simulink model "GNC2026W"  (R2024b)
settings: Solver=ode4  StartTime=0.0  StopTime=tsim  FixedStep=baseRate
values from neighbouring files (symbols this model uses):
  a = 1    [Run_Initializer.m]    (also in UKFoptimization.m)
  a1 = 0.236940    (= 0.23694)    [DrawARM.m]    (also in Run_Initializer.m = 2)
  a2 = 0.281536    [DrawARM.m]    (also in Run_Initializer.m = 2)
  a3 = 0.0621    [DrawARM.m]    (also in Run_Initializer.m = 2)
  A_c = eye(3)    [Run_Initializer.m]
  alpha = diag([a1; a2; a3])    [Run_Initializer.m]    (also in overlapping_trajectories.m = alpha_values1(ii); plotTrajectory.m = alpha_values(ii); plotfig.m = alpha_values(ii))
  b = 2    [Run_Initializer.m]    (also in UKFoptimization.m)
  b0 = 0.230400    (= 0.2304)    [DrawARM.m]
  b1 = 0.078980    (= 0.07898)    [DrawARM.m]
  b2 = 0.070384    [DrawARM.m]
  b3 = 0.070685    [DrawARM.m]
  CVrate = 1/5    (= 0.2)    [Run_Initializer.m]
  dt = baseRate    [Run_Initializer.m]    (also in UKFoptimization.m = 0.05; rms_plots.m = median(diff(tA)))
  F_u = zeros(3,1)    [Run_Initializer.m]
  fNum = 1    [Run_Initializer.m]
  gamma = r - (excess + shrink + bracketwidth)    (= 0.05023)    [DrawSpacecraft.m]    (also in Run_Initializer.m = diag([g1; g2; g3]))
  Gamma1_el = 0.12    [Run_Initializer.m]
  Gamma1_sh = 0.005    [Run_Initializer.m]
  Gamma1_wr = 0.025    [Run_Initializer.m]
  Gamma2_el = 5    [Run_Initializer.m]
  Gamma2_sh = 5    [Run_Initializer.m]
  Gamma2_wr = 5    [Run_Initializer.m]
  Gamma3_el = 10    [Run_Initializer.m]
  Gamma3_sh = 40    [Run_Initializer.m]
  Gamma3_wr = 40    [Run_Initializer.m]
  Gamma4_el = 0.039    [Run_Initializer.m]
  Gamma4_sh = 0.015    [Run_Initializer.m]
  Gamma4_wr = 0.029    [Run_Initializer.m]
  Gamma5_el = 800    [Run_Initializer.m]
  Gamma5_sh = 800    [Run_Initializer.m]
  Gamma5_wr = 800    [Run_Initializer.m]
  Gamma6_el = 0.000001    (= 1e-06)    [Run_Initializer.m]
  Gamma6_sh = 0.005    [Run_Initializer.m]
  Gamma6_wr = 0.02    [Run_Initializer.m]
  k = 5    [Run_Initializer.m]    (also in UKFoptimization.m)
  Kd_elarm = 0.8    [Run_Initializer.m]
  Kd_sharm = 1.0    (= 1)    [Run_Initializer.m]
  Kd_wrarm = 0.6    [Run_Initializer.m]
  Kp_elarm = 1.2    [Run_Initializer.m]
  Kp_sharm = 1.5    [Run_Initializer.m]
  Kp_wrarm = 1.0    (= 1)    [Run_Initializer.m]
  Mc_inv = inv(M_c)    [Run_Initializer.m]
  Phi = 73.2749*pi/180    (= 1.27888826407)    [DrawARM.m]
  PWMFreq = 5    [Run_Initializer.m]
  R = [cos(theta) -sin(theta) ... (first row only)    [Run_Initializer.m]    (also in UKFoptimization.m = diag([rx, rx, rt]))
  sep1 = 0.60    (= 0.6)    [Run_Initializer.m]
  sep2 = 0.30    (= 0.3)    [Run_Initializer.m]
  sep3 = 0.30    (= 0.3)    [Run_Initializer.m]
  Tz_lim_elarm = .1    (= 0.1)    [Run_Initializer.m]
  Tz_lim_sharm = .1    (= 0.1)    [Run_Initializer.m]
  Tz_lim_wrarm = .1    (= 0.1)    [Run_Initializer.m]
  VISinLoop = 1    [Run_Initializer.m]
  X1_blk = 0.4    [Run_Initializer.m]
  X2_blk = 0.4    [Run_Initializer.m]
  X3_blk = 0.4    [Run_Initializer.m]
  Y1_blk = 0.4    [Run_Initializer.m]
  Y2_blk = 0.4    [Run_Initializer.m]
  Y3_blk = 0.4    [Run_Initializer.m]
undefined symbols (not defined in the file or in its folder): baseRate, dataRate, DiscIntNeverNeededParam, drop_states_ARM, drop_states_BLACK, drop_states_BLUE, drop_states_RED, F_red_X_nominal, F_red_Y_nominal, F_thrusters_BLACK, F_thrusters_BLUE, F_thrusters_RED, home_states_BLACK, home_states_BLUE, home_states_RED, IBLACK, IBLUE, IDIST, IEE, init_states_BLACK, init_states_BLUE, init_states_RED, IPROX, IRED, K_BLACK, K_BLUE, K_RED, Kd_tb, Kd_tblue, Kd_tr, Kd_xb, Kd_xblue, Kd_xr, Kd_yb, Kd_yblue, Kd_yr, Kp_tb, Kp_tblue, Kp_tr, Kp_xb, Kp_xblue, Kp_xr, Kp_yb, Kp_yblue, Kp_yr, mBLACK, mBLUE, mDIST, mEE, mPROX, mRED, Phase0_End, Phase1_End, Phase2_End, Phase3_End, Phase3_SubPhase1_End, Phase3_SubPhase2_End, Phase3_SubPhase3_End, Phase3_SubPhase4_End, Phase4_End ... (+10)
libraries: simulink x30, nvidiaSharedBlocks x20, MainLibrary x5, dspinverses x3, commrandsrc3 x1, nvidiaIMUSensorslib x1
(part 8 of 9)

== matlab function GNC2026W/Simulate Plant Dynamics/RED and ARM Dynamics/RED + ARM/Coriolis Function1 ==
  data: a1 parameter; a2 parameter; a3 parameter; b0 parameter; b1 parameter; b2 parameter; mPROX parameter; mDIST parameter; mEE parameter; Phi parameter; CoriolisS output; x input
function CoriolisS = CoriolisFunc3LINK(a1,a2,a3,b0,b1,b2,mPROX,mDIST,mEE,Phi,x)
%CORIOLISFUNC3LINK
%    CORIOLISS = CORIOLISFUNC3LINK(A1,A2,A3,B0,B1,B2,mPROX,mDIST,mEE,PHI,Q0,Q1,Q2,Q3,Q0_DOT,Q1_DOT,Q2_DOT,Q3_DOT)

%    This function was generated by the Symbolic Math Toolbox version 8.0.
%    05-Nov-2017 11:48:44

q0 = x(3);
q1 = x(4);
q2 = x(5);
q3 = x(6);

q0_dot = x(9);
q1_dot = x(10);
q2_dot = x(11);
q3_dot = x(12);

t2 = a1+b1;
t3 = a1.*mPROX;
t4 = mDIST.*t2;
t5 = mEE.*t2;
t6 = t3+t4+t5;
t7 = a2.*mDIST;
t8 = a2+b2;
t9 = mEE.*t8;
t10 = t7+t9;
t11 = pi.*(1.0./2.0);
t12 = q0_dot.*t6;
t13 = q1_dot.*t6;
t14 = q0+q1+t11;
t15 = cos(t14);
t16 = t12+t13;
t17 = q0_dot.*t10;
t18 = q1_dot.*t10;
t19 = q2_dot.*t10;
t20 = q0+q1+q2+t11;
t21 = cos(t20);
t22 = t17+t18+t19;
t23 = a3.*mEE.*q0_dot;
t24 = a3.*mEE.*q1_dot;
t25 = a3.*mEE.*q2_dot;
t26 = a3.*mEE.*q3_dot;
t27 = q0+q1+q2+q3+t11;
t28 = cos(t27);
t29 = t23+t24+t25+t26;
t30 = b0.*mPROX;
t31 = b0.*mDIST;
t32 = b0.*mEE;
t33 = t30+t31+t32;
t34 = (pi/2-Phi)+q0;
t35 = sin(t14);
t36 = sin(t20);
t37 = sin(t27);
t38 = q0_dot+q1_dot+q2_dot+q3_dot;
t39 = q0+q1+q2+q3;
t40 = a1.*b0.*mPROX.*q1_dot;
t41 = a1.*b0.*mDIST.*q1_dot;
t42 = a1.*b0.*mEE.*q1_dot;
t43 = b0.*b1.*mDIST.*q1_dot;
t44 = b0.*b1.*mEE.*q1_dot;
t45 = (pi/2-Phi)-q1;
t46 = cos(t45);
t47 = a2.*b0.*mDIST.*q1_dot;
t48 = a2.*b0.*mDIST.*q2_dot;
t49 = a2.*b0.*mEE.*q1_dot;
t50 = a2.*b0.*mEE.*q2_dot;
t51 = b0.*b2.*mEE.*q1_dot;
t52 = b0.*b2.*mEE.*q2_dot;
t53 = -(pi/2-Phi)+q1+q2;
t54 = cos(t53);
t55 = a3.*b0.*mEE.*q1_dot;
t56 = a3.*b0.*mEE.*q2_dot;
t57 = a3.*b0.*mEE.*q3_dot;
t58 = -(pi/2-Phi)+q1+q2+q3;
t59 = cos(t58);
t60 = a2.*b1.*mDIST.*q2_dot;
t61 = a1.*b2.*mEE.*q2_dot;
t62 = a2.*b1.*mEE.*q2_dot;
t63 = b1.*b2.*mEE.*q2_dot;
t64 = a1.*a2.*mDIST.*q2_dot;
t65 = a1.*a2.*mEE.*q2_dot;
t66 = sin(q2);
t67 = t60+t61+t62+t63+t64+t65;
t68 = a3.*b2.*mEE.*q3_dot;
t69 = a2.*a3.*mEE.*q3_dot;
t70 = sin(q3);
t71 = t68+t69;
t72 = a3.*b1.*mEE.*q2_dot;
t73 = a3.*b1.*mEE.*q3_dot;
t74 = a1.*a3.*mEE.*q2_dot;
t75 = a1.*a3.*mEE.*q3_dot;
t76 = q2+q3;
t77 = sin(t76);
t78 = t72+t73+t74+t75;
t79 = a2.*b0.*mDIST.*q0_dot;
t80 = a2.*b0.*mEE.*q0_dot;
t81 = b0.*b2.*mEE.*q0_dot;
t82 = t47+t48+t49+t50+t51+t52+t79+t80+t81;
t83 = a3.*b0.*mEE.*q0_dot;
t84 = t55+t56+t57+t83;
t85 = a1.*b0.*mPROX.*q0_dot;
t86 = a1.*b0.*mDIST.*q0_dot;
t87 = a1.*b0.*mEE.*q0_dot;
t88 = b0.*b1.*mDIST.*q0_dot;
t89 = b0.*b1.*mEE.*q0_dot;
t90 = a2.*b1.*mDIST.*q0_dot;
t91 = a1.*b2.*mEE.*q0_dot;
t92 = a2.*b1.*mDIST.*q1_dot;
t93 = a2.*b1.*mEE.*q0_dot;
t94 = a1.*b2.*mEE.*q1_dot;
t95 = a2.*b1.*mEE.*q1_dot;
t96 = b1.*b2.*mEE.*q0_dot;
t97 = b1.*b2.*mEE.*q1_dot;
t98 = a1.*a2.*mDIST.*q0_dot;
t99 = a1.*a2.*mDIST.*q1_dot;
t100 = a1.*a2.*mEE.*q0_dot;
t101 = a1.*a2.*mEE.*q1_dot;
t102 = t60+t61+t62+t63+t64+t65+t90+t91+t92+t93+t94+t95+t96+t97+t98+t99+t100+t101;
t103 = a3.*b1.*mEE.*q0_dot;
t104 = a3.*b1.*mEE.*q1_dot;
t105 = a1.*a3.*mEE.*q0_dot;
t106 = a1.*a3.*mEE.*q1_dot;
t107 = t72+t73+t74+t75+t103+t104+t105+t106;
t108 = t79+t80+t81;
t109 = t54.*t108;
t110 = t59.*t83;
t111 = t90+t91+t92+t93+t94+t95+t96+t97+t98+t99+t100+t101;
t112 = t66.*t111;
t113 = t103+t104+t105+t106;
t114 = t77.*t113;
t115 = a2.*q0_dot;
t116 = a2.*q1_dot;
t117 = a2.*q2_dot;
t118 = b2.*q0_dot;
t119 = b2.*q1_dot;
t120 = b2.*q2_dot;
t121 = t115+t116+t117+t118+t119+t120;
t122 = a3.*mEE.*t70.*t121;
t123 = a1.*q0_dot;
t124 = a1.*q1_dot;
t125 = b1.*q0_dot;
t126 = b1.*q1_dot;
t127 = t123+t124+t125+t126;
t128 = a3.*mEE.*t77.*t127;
CoriolisS = reshape([0.0,0.0,0.0,0.0,0.0,0.0,0.0,0.0,0.0,0.0,0.0,0.0,-t15.*t16-t21.*t22-t28.*t29-q0_dot.*t33.*cos(t34),-t16.*t35-t22.*t36-t29.*t37-q0_dot.*t33.*sin(t34),-t66.*t67-t70.*t71-t77.*t78-t46.*(t40+t41+t42+t43+t44)-t59.*(t55+t56+t57)-t54.*(t47+t48+t49+t50+t51+t52),t109+t110-t66.*t67-t70.*t71-t77.*t78+t46.*(t85+t86+t87+t88+t89),t109+t110+t112+t114-t70.*t71,t110+t122+t128,-t15.*t16-t21.*t22-t28.*t29,-t16.*t35-t22.*t36-t29.*t37,-t66.*t67-t54.*t82-t70.*t71-t59.*t84-t77.*t78-t46.*(t40+t41+t42+t43+t44+t85+t86+t87+t88+t89),-t66.*t67-t70.*t71-t77.*t78,t112+t114-t70.*t71,t122+t128,-t21.*t22-t28.*t29,-t22.*t36-t29.*t37,-t54.*t82-t70.*t71-t59.*t84-t66.*t102-t77.*t107,-t70.*t71-t66.*t102-t77.*t107,-a3.*mEE.*q3_dot.*t8.*t70,a3.*mEE.*t8.*t70.*(q0_dot+q1_dot+q2_dot),a3.*mEE.*t38.*sin(t39),-a3.*mEE.*t38.*cos(t39),-a3.*b0.*mEE.*t38.*t59-a3.*mEE.*t8.*t38.*t70-a3.*mEE.*t2.*t38.*t77,-a3.*mEE.*t8.*t38.*t70-a3.*mEE.*t2.*t38.*t77,-a3.*mEE.*t8.*t38.*t70,0.0],[6,6]);
end

== matlab function GNC2026W/Simulate Plant Dynamics/BLACK Dynamics/Data @ Measurement Rate/Calculate True Time Step/MATLAB Function ==
  data: dt input; dt_out output; dataRate input
function dt_out = CheckforInvalidTime(dt, dataRate)

    if dt <= 0

        dt_out = dataRate;

    else

        dt_out = dt;

    end


end

== matlab function GNC2026W/Simulate Plant Dynamics/RED and ARM Dynamics/RED + ARM/Inertia Function 1 ==
  data: mRED parameter; IRED parameter; Phi parameter; b0 parameter; a1 parameter; b1 parameter; a2 parameter; b2 parameter; a3 parameter; b3 parameter; mPROX parameter; mDIST parameter; mEE parameter; IPROX parameter; IDIST parameter; InertiaS output; x input; IEE parameter
function InertiaS = InertiaFunc3LINK(mRED, IRED, Phi, b0, a1, b1, a2, b2, a3, b3, mPROX, mDIST, mEE, IPROX, IDIST, x, IEE)

    q0 = x(3);
    q1 = x(4);
    q2 = x(5);
    q3 = x(6);
    
    t2 = a1+b1;
    t3 = a1.*mPROX;
    t4 = mDIST.*t2;
    t5 = mEE.*t2;
    t6 = q0+q1;
    t7 = cos(t6);
    t8 = t3+t4+t5;
    t9 = a2.*mDIST;
    t10 = a2+b2;
    t11 = mEE.*t10;
    t12 = q0+q1+q2;
    t13 = cos(t12);
    t14 = t9+t11;
    t15 = q0+q1+q2+q3;
    t16 = cos(t15);
    t17 = mRED+mPROX+mDIST+mEE;
    t18 = b0.*mPROX;
    t19 = b0.*mDIST;
    t20 = b0.*mEE;
    t21 = t18+t19+t20;
    t22 = (pi/2-Phi)+q0;
    t23 = sin(t6);
    t24 = sin(t12);
    t25 = sin(t15);
    t26 = a2.*mEE;
    t27 = b2.*mEE;
    t28 = t9+t26+t27;
    t29 = sin(t22);
    t86 = t7.*t8;
    t87 = t13.*t14;
    t88 = a3.*mEE.*t16;
    t30 = -t86-t87-t88-t21.*t29;
    t31 = cos(t22);
    t32 = t21.*t31;
    t89 = t8.*t23;
    t90 = t14.*t24;
    t91 = a3.*mEE.*t25;
    t33 = t32-t89-t90-t91;
    t34 = a1.^2;
    t35 = a2.^2;
    t36 = b0.^2;
    t37 = b1.^2;
    t38 = a1.*a2.*mDIST.*2.0;
    t39 = a1.*a2.*mEE.*2.0;
    t40 = a2.*b1.*mDIST.*2.0;
    t41 = a1.*b2.*mEE.*2.0;
    t42 = a2.*b1.*mEE.*2.0;
    t43 = b1.*b2.*mEE.*2.0;
    t44 = t38+t39+t40+t41+t42+t43;
    t45 = cos(q2);
    t46 = t44.*t45;
    t47 = a2.*a3.*mEE.*2.0;
    t48 = a3.*b2.*mEE.*2.0;
    t49 = t47+t48;
    t50 = cos(q3);
    t51 = t49.*t50;
    t52 = a1.*a3.*mEE.*2.0;
    t53 = a3.*b1.*mEE.*2.0;
    t54 = t52+t53;
    t55 = q2+q3;
    t56 = cos(t55);
    t57 = t54.*t56;
    t58 = (pi/2-Phi)-q1;
    t59 = sin(t58);
    t60 = -(pi/2-Phi)+q1+q2;
    t61 = sin(t60);
    t62 = -(pi/2-Phi)+q1+q2+q3;
    t63 = sin(t62);
    t64 = mPROX.*t34;
    t65 = mDIST.*t34;
    t66 = mEE.*t34;
    t67 = mDIST.*t35;
    t68 = mEE.*t35;
    t69 = a3.^2;
    t70 = mEE.*t69;
    t71 = mDIST.*t37;
    t72 = mEE.*t37;
    t73 = b2.^2;
    t74 = mEE.*t73;
    t75 = a1.*b1.*mDIST.*2.0;
    t76 = a1.*b1.*mEE.*2.0;
    t77 = a2.*b2.*mEE.*2.0;
    t78 = a2.*b0.*mDIST;
    t79 = a2.*b0.*mEE;
    t80 = b0.*b2.*mEE;
    t81 = t78+t79+t80;
    t82 = a1.*a3.*mEE;
    t83 = a3.*b1.*mEE;
    t84 = t82+t83;
    t85 = t56.*t84;
    t92 = a1.*b0.*mPROX;
    t93 = a1.*b0.*mDIST;
    t94 = a1.*b0.*mEE;
    t95 = b0.*b1.*mDIST;
    t96 = b0.*b1.*mEE;
    t97 = t92+t93+t94+t95+t96;
    t98 = t59.*t97;
    t112 = t61.*t81;
    t113 = a3.*b0.*mEE.*t63;
    t99 = IPROX+IDIST+IEE+t46+t51+t57+t64+t65+t66+t67+t68+t70+t71+t72+t74+t75+t76+t77+t98-t112-t113;
    t100 = a1.*a2.*mDIST;
    t101 = a1.*a2.*mEE;
    t102 = a2.*b1.*mDIST;
    t103 = a1.*b2.*mEE;
    t104 = a2.*b1.*mEE;
    t105 = b1.*b2.*mEE;
    t106 = t100+t101+t102+t103+t104+t105;
    t107 = t45.*t106;
    t108 = a2.*a3.*mEE;
    t109 = a3.*b2.*mEE;
    t110 = t108+t109;
    t111 = t50.*t110;
    t114 = IDIST+IEE+t51+t67+t68+t70+t74+t77+t85+t107;
    t115 = IEE+t70+t85+t111;
    t116 = IEE+t70+t111;
    InertiaS = reshape([t17,0.0,t30,-t86-t87-t88,-t88-t13.*t28,-t88,0.0,t17,t33,-t89-t90-t91,-t91-t24.*t28,-t91,t30,t33,IRED+IPROX+IDIST+IEE+t46+t51+t57+t64+t65+t66+t67+t68+t70+t71+t72+t74+t75+t76+t77+t59.*(a1.*b0.*mPROX.*2.0+a1.*b0.*mDIST.*2.0+a1.*b0.*mEE.*2.0+b0.*b1.*mDIST.*2.0+b0.*b1.*mEE.*2.0)+mPROX.*t36+mDIST.*t36+mEE.*t36-t61.*(a2.*b0.*mDIST.*2.0+a2.*b0.*mEE.*2.0+b0.*b2.*mEE.*2.0)-a3.*b0.*mEE.*t63.*2.0,t99,IDIST+IEE+t51+t67+t68+t70+t74+t77+t85+t107-t112-t113,IEE+t70+t85+t111-t113,-t7.*t8-t13.*t14-a3.*mEE.*t16,-t8.*t23-t14.*t24-a3.*mEE.*t25,t99,IPROX+IDIST+IEE+t46+t51+t57+t64+t65+t66+t67+t68+t70+t71+t72+t74+t75+t76+t77,t114,t115,-t13.*t28-a3.*mEE.*t16,-t24.*t28-a3.*mEE.*t25,IDIST+IEE+t51+t67+t68+t70+t74+t77+t85+t107-t61.*t81-a3.*b0.*mEE.*t63,t114,IDIST+IEE+t51+t67+t68+t70+t74+t77,t116,-a3.*mEE.*t16,-a3.*mEE.*t25,IEE+t70+t85+t111-a3.*b0.*mEE.*t63,t115,t116,IEE+t70],[6,6]);
end

== matlab function GNC2026W/Simulate Plant Dynamics/BLUE Dynamics/Calculated & Store Measured States/Subsystem1/Enabled Subsystem/MATLAB Function ==
  data: y input; dy output; dt input; tau input; ema_prev input; ema output
function [dy, ema] = realtime_derivative_ema(y, dt, tau, ema_prev)
    % Compute smoothed derivative using Exponential Moving Average
    %
    % Inputs:
    %   y        : Current measurement
    %   dt       : Time step
    %   tau      : Time constant for EMA filter (larger = more smoothing)
    %   ema_prev : Previous EMA value
    %
    % Outputs:
    %   dy  : Smoothed derivative estimate
    %   ema : Updated EMA value
    
    % Calculate smoothing factor from time constant
    alpha = 1 - exp(-dt ./ tau);
    
    % Update Exponential Moving Average
    ema = alpha .* y + (1 - alpha) .* ema_prev;
    
    % Compute derivative using finite difference on smoothed values
    dy = (ema - ema_prev) ./ dt;
end

== matlab function GNC2026W/Simulate Plant Dynamics/BLACK Dynamics/Dynamics Model for BLACK/MATLAB Function ==
  data: control_inputs input; x_ddot output; mBLACK parameter; IBLACK parameter
function x_ddot = BLACK_dynamics(control_inputs, mBLACK, IBLACK)

%#codegen
% Fully define the size of x_ddot() for code generation:
x_ddot     = zeros(3,1);

% Extract the control inputs from the control_input vector:
Fx        = control_inputs(1);              % [N]
Fy        = control_inputs(2);              % [N]
Tz        = control_inputs(3);              % [N.m]

% Calculate the state acceleration vector:
x_ddot(1) = Fx/mBLACK;                      % [m/s^2]
x_ddot(2) = Fy/mBLACK;                      % [m/s^2]
x_ddot(3) = Tz/IBLACK;                      % [rad/s^2]

end

== matlab function GNC2026W/Simulate Plant Dynamics/BLUE Dynamics/BLUE  Dynamics Model/MATLAB Function ==
  data: control_inputs input; x_ddot output; mBLUE parameter; IBLUE parameter
function x_ddot = BLUE_dynamics(control_inputs, mBLUE, IBLUE)%#codegen
% Fully define the size of x_ddot() for code generation:
x_ddot     = zeros(3,1);

% Extract the control inputs from the control_input vector:
Fx        = control_inputs(1);              % [N]
Fy        = control_inputs(2);              % [N]
Tz        = control_inputs(3);              % [N.m]

% Calculate the state acceleration vector:
x_ddot(1) = Fx/mBLUE;                      % [m/s^2]
x_ddot(2) = Fy/mBLUE;                      % [m/s^2]
x_ddot(3) = Tz/IBLUE;                      % [rad/s^2]

end

== matlab function GNC2026W/Gyro.//Accel. Code/Log Gyro//Accel/Parse IMU Data ==
  data: WhoAmI input; RED_IMU_Ax output; IMU_Ax input; IMU_Ay input; IMU_Gz input; RED_IMU_Ay output; RED_IMU_Gz output; BLACK_IMU_Ax output; BLACK_IMU_Ay output; BLACK_IMU_Gz output; BLUE_IMU_Ax output; BLUE_IMU_Ay output; BLUE_IMU_Gz output
function [RED_IMU_Ax, RED_IMU_Ay, RED_IMU_Gz, BLACK_IMU_Ax, BLACK_IMU_Ay, BLACK_IMU_Gz, BLUE_IMU_Ax, BLUE_IMU_Ay, BLUE_IMU_Gz] = ParseIMUData(WhoAmI, IMU_Ax, IMU_Ay, IMU_Gz)

    if WhoAmI == 1 % This is RED

        RED_IMU_Ax = IMU_Ax;
        RED_IMU_Ay = IMU_Ay;
        RED_IMU_Gz = IMU_Gz;
        BLACK_IMU_Ax = 0;
        BLACK_IMU_Ay = 0;
        BLACK_IMU_Gz = 0;
        BLUE_IMU_Ax = 0;
        BLUE_IMU_Ay = 0;
        BLUE_IMU_Gz = 0;

    elseif WhoAmI == 2 % This is BLACK

        RED_IMU_Ax = 0;
        RED_IMU_Ay = 0;
        RED_IMU_Gz = 0;
        BLACK_IMU_Ax = IMU_Ax;
        BLACK_IMU_Ay = IMU_Ay;
        BLACK_IMU_Gz = IMU_Gz;
        BLUE_IMU_Ax = 0;
        BLUE_IMU_Ay = 0;
        BLUE_IMU_Gz = 0;

    elseif WhoAmI == 3 % This is BLUE

        RED_IMU_Ax = 0;
        RED_IMU_Ay = 0;
        RED_IMU_Gz = 0;
        BLACK_IMU_Ax = 0;
        BLACK_IMU_Ay = 0;
        BLACK_IMU_Gz = 0;
        BLUE_IMU_Ax = IMU_Ax;
        BLUE_IMU_Ay = IMU_Ay;
        BLUE_IMU_Gz = IMU_Gz;

    else 

        RED_IMU_Ax = 0;
        RED_IMU_Ay = 0;
        RED_IMU_Gz = 0;
        BLACK_IMU_Ax = 0;
        BLACK_IMU_Ay = 0;
        BLACK_IMU_Gz = 0;
        BLUE_IMU_Ax = 0;
        BLUE_IMU_Ay = 0;
        BLUE_IMU_Gz = 0;       

    end

end

== matlab function GNC2026W/Simulate Plant Dynamics/BLUE Dynamics/Calculated & Store Measured States/Subsystem2/Enabled Subsystem/MATLAB Function ==
  data: y input; dy output; dt input; tau input; ema_prev input; ema output
function [dy, ema] = realtime_derivative_ema(y, dt, tau, ema_prev)
    % Compute smoothed derivative using Exponential Moving Average
    %
    % Inputs:
    %   y        : Current measurement
    %   dt       : Time step
    %   tau      : Time constant for EMA filter (larger = more smoothing)
    %   ema_prev : Previous EMA value
    %
    % Outputs:
    %   dy  : Smoothed derivative estimate
    %   ema : Updated EMA value
    
    % Calculate smoothing factor from time constant
    alpha = 1 - exp(-dt ./ tau);
    
    % Update Exponential Moving Average
    ema = alpha .* y + (1 - alpha) .* ema_prev;
    
    % Compute derivative using finite difference on smoothed values
    dy = (ema - ema_prev) ./ dt;
end

== matlab function GNC2026W/Simulate Plant Dynamics/BLUE Dynamics/Data @ Measurement Rate/Calculate True Time Step/MATLAB Function ==
  data: dt input; dt_out output; dataRate input
function dt_out = CheckforInvalidTime(dt, dataRate)

    if dt <= 0

        dt_out = dataRate;

    else

        dt_out = dt;

    end


end

== matlab function GNC2026W/Thruster Control Code/Change BLUE Behavior/Calculate Duty Cycle/MATLAB Function5 ==
  data: H_final output; u_desired input; duty_cycles output; x0 input; thruster_dist2CG_RED parameter; F_red_X_nominal parameter; F_red_Y_nominal parameter; max_iters parameter; tol parameter
function [H_final, duty_cycles] = optimize_duty_cycle_with_decay( ...
    u_desired, x0, thruster_dist2CG_RED, F_red_X_nominal, F_red_Y_nominal, max_iters, tol)
    %OPTIMIZE_DUTY_CYCLE_WITH_DECAY 
    %   Iteratively optimizes thruster duty cycles while updating thrust decay.
    %
    %   Inputs:
    %       u_desired           - Desired force/torque vector [Fx; Fy; M] (3x1)
    %       x0                  - Initial guess for duty cycles (8x1)
    %       thruster_dist2CG_RED- Distances of thrusters from CG (vector, mm)
    %       F_red_X_nominal     - Nominal X-direction thruster force (scalar, N)
    %       F_red_Y_nominal     - Nominal Y-direction thruster force (scalar, N)
    %       max_iters           - Maximum optimization iterations
    %       tol                 - Convergence tolerance (on duty cycles)
    %
    %   Outputs:
    %       H_final     - Final H-matrix including thrust decay (3x8)
    %       duty_cycles - Optimized duty cycles (8x1)
    %

    % ---------------------------
    % Initialization
    % ---------------------------
    num_thrusters      = length(x0); %#ok<NASGU> % reserved if needed later
    duty_cycles        = x0;                     % current solution
    thrust_decay_factor = 1;                     % initial decay
    prev_duty_cycles   = duty_cycles + 2*tol;    % force first iteration

    % ---------------------------
    % Iterative optimization
    % ---------------------------
    for iter = 1:max_iters
        % Build system matrix H with current decay factor
        H = MakeHWithDecay(thruster_dist2CG_RED, F_red_X_nominal, ...
                           thrust_decay_factor, F_red_Y_nominal);

        % Solve constrained least squares (box constraints: 0 ≤ x ≤ 1)
        duty_cycles = custom_constrained_least_squares(H, u_desired, duty_cycles);

        % Update decay factor based on the current duty cycles
        [thrust_decay_factor, ~] = check_thrust_decay(duty_cycles);

        % Check convergence (∞-norm difference)
        if norm(duty_cycles - prev_duty_cycles, Inf) < tol
            H_final = MakeHWithDecayRecalculateForce(thruster_dist2CG_RED, ...
                        F_red_X_nominal, thrust_decay_factor, F_red_Y_nominal);
            return;
        end

        % Update reference for next iteration
        prev_duty_cycles = duty_cycles;
    end

    % If not converged within max_iters, return final H with last decay
    H_final = MakeHWithDecayRecalculateForce(thruster_dist2CG_RED, ...
                F_red_X_nominal, thrust_decay_factor, F_red_Y_nominal);
end


% ========================================================================
% Custom Constrained Least Squares Solver
% ========================================================================
function x_opt = custom_constrained_least_squares(H, b, x0)
    %CUSTOM_CONSTRAINED_LEAST_SQUARES
    %   Solves min_x ||H*x - b||^2 subject to 0 <= x <= 1
    %   using projected gradient descent with backtracking line search.
    %
    %   Inputs:
    %       H   - System matrix (3x8)
    %       b   - Desired vector (3x1)
    %       x0  - Initial guess (8x1)
    %
    %   Output:
    %       x_opt - Optimal duty cycle vector (8x1)

    % Parameters
    max_iterations = 100;
    tolerance      = 1e-6;
    alpha          = 0.01;  % initial step size
    beta           = 0.5;   % backtracking factor

    % Initialization
    x      = x0;
    x_prev = x0 + 2*tolerance;

    % Precompute matrices
    HtH = H' * H;
    Htb = H' * b;

    for iter = 1:max_iterations
        % Gradient of ||H*x - b||^2
        gradient = 2 * (HtH*x - Htb);

        % Store objective for comparison
        current_obj = norm(H*x - b)^2;

        % Backtracking line search
        step_size = alpha;
        for ls_iter = 1:20
            x_new = x - step_size * gradient;
            x_new = max(0, min(1, x_new)); % project into [0,1]

            new_obj = norm(H*x_new - b)^2;
            if new_obj < current_obj
                break; % accept step
            else
                step_size = step_size * beta;
            end
        end

        % Update
        x = x_new;

        % Convergence check
        if norm(x - x_prev) < tolerance
            break;
        end

        % Adaptive step size tuning
        if iter > 1 && new_obj < current_obj
            alpha = min(alpha * 1.1, 0.1); % speed up if progress
        else
            alpha = alpha * 0.9;           % slow down otherwise
        end

        % Store for next iteration
        x_prev = x;
    end

    x_opt = x;
end


% ========================================================================
% Construct H-matrix (with decay factor)
% ========================================================================
function H = MakeHWithDecay(thruster_dist2CG, F_X_nominal, thrust_decay_factor, F_Y_nominal)
    %MAKEHWITHDECAY
    %   Builds the H matrix that maps thruster duty cycles to [Fx; Fy; M],
    %   applying thrust decay.
    %
    %   Outputs H as (3x8)

    % Convert thruster arm distances to meters
    adjusted_dist = thruster_dist2CG / 1000;

    % Thruster directions (X, Y, and moment arm)
    Vec1 = [-1; -1;  0;  0;  1;  1;  0;  0]; % X
    Vec2 = [ 0;  0;  1;  1;  0;  0; -1; -1]; % Y
    Vec3 = adjusted_dist;                    % moment (Z)

    Mat1 = [Vec1, Vec2, Vec3]';

    % Thruster forces (scaled by decay)
    F_thrusters = [F_X_nominal; F_X_nominal; ...
                   F_Y_nominal; F_Y_nominal; ...
                   F_X_nominal; F_X_nominal; ...
                   F_Y_nominal; F_Y_nominal] * thrust_decay_factor;

    % Build diagonal scaling
    Mat2 = diag(F_thrusters / 2);

    % Final mapping
    H = Mat1 * Mat2;
end


% ========================================================================
% Construct H-matrix (recalculate full force with decay)
% ========================================================================
function H = MakeHWithDecayRecalculateForce(thruster_dist2CG, F_X_nominal, thrust_decay_factor, F_Y_nominal)
    %MAKEHWITHDECAYRECALCULATEFORCE
    %   Same as MakeHWithDecay but applies full nominal force scaling.

    adjusted_dist = thruster_dist2CG / 1000;

    Vec1 = [-1; -1;  0;  0;  1;  1;  0;  0];
    Vec2 = [ 0;  0;  1;  1;  0;  0; -1; -1];
    Vec3 = adjusted_dist;

    Mat1 = [Vec1, Vec2, Vec3]';

    F_thrusters = [F_X_nominal; F_X_nominal; ...
                   F_Y_nominal; F_Y_nominal; ...
                   F_X_nominal; F_X_nominal; ...
                   F_Y_nominal; F_Y_nominal] * thrust_decay_factor;

    Mat2 = diag(F_thrusters);

    H = Mat1 * Mat2;
end


% ========================================================================
% Thrust Decay Update Rule
% ========================================================================
function [thrust_decay_factor, count] = check_thrust_decay(PWMs)
    %CHECK_THRUST_DECAY
    %   Updates thrust decay factor based on average duty cycle.
    %
    %   Inputs:
    %       PWMs - Duty cycle vector (8x1)
    %
    %   Outputs:
    %       thrust_decay_factor - Adjusted decay factor (scalar)
    %       count               - Number of active thrusters

    % Normalize if needed
    if max(PWMs) > 1
        PWMs = PWMs / max(PWMs);
    end
    
    % Active thrusters
    count = sum(PWMs > 0);
    
    % Mean duty cycle (only active thrusters)
    avg_duty = sum(max(PWMs, 0)) / max(count, 1);
    
    % Update rule (piecewise)
    if avg_duty < 0.3 || count == 0
        thrust_decay_factor = 1;
    else
        thrust_decay_factor = max(0.6 - 2*avg_duty + 1, 0.5);
    end
end

== matlab function GNC2026W/PhaseSpace Camera Code/Use Hardware to Obtain States/Store RED Data/Subsystem2/Enabled Subsystem/MATLAB Function ==
  data: y input; dy output; dt input; tau input; ema_prev input; ema output
function [dy, ema] = realtime_derivative_ema(y, dt, tau, ema_prev)
    % Compute smoothed derivative using Exponential Moving Average
    %
    % Inputs:
    %   y        : Current measurement
    %   dt       : Time step
    %   tau      : Time constant for EMA filter (larger = more smoothing)
    %   ema_prev : Previous EMA value
    %
    % Outputs:
    %   dy  : Smoothed derivative estimate
    %   ema : Updated EMA value
    
    % Calculate smoothing factor from time constant
    alpha = 1 - exp(-dt ./ tau);
    
    % Update Exponential Moving Average
    ema = alpha .* y + (1 - alpha) .* ema_prev;
    
    % Compute derivative using finite difference on smoothed values
    dy = (ema - ema_prev) ./ dt;
end

== matlab function GNC2026W/PhaseSpace Camera Code/Use Hardware to Obtain States/Store BLACK Data/Calculate True Time Step/MATLAB Function ==
  data: dt input; dt_out output; dataRate input
function dt_out = CheckforInvalidTime(dt, dataRate)

    if dt <= 0

        dt_out = dataRate;

    else

        dt_out = dt;

    end


end

== matlab function GNC2026W/PhaseSpace Camera Code/Use Hardware to Obtain States/Store RED Data/Calculate True Time Step/MATLAB Function ==
  data: dt input; dt_out output; dataRate input
function dt_out = CheckforInvalidTime(dt, dataRate)

    if dt <= 0

        dt_out = dataRate;

    else

        dt_out = dt;

    end


end

== matlab function GNC2026W/PhaseSpace Camera Code/Use Hardware to Obtain States/Store BLACK Data/Subsystem1/Enabled Subsystem/MATLAB Function ==
  data: y input; dy output; dt input; tau input; ema_prev input; ema output
function [dy, ema] = realtime_derivative_ema(y, dt, tau, ema_prev)
    % Compute smoothed derivative using Exponential Moving Average
    %
    % Inputs:
    %   y        : Current measurement
    %   dt       : Time step
    %   tau      : Time constant for EMA filter (larger = more smoothing)
    %   ema_prev : Previous EMA value
    %
    % Outputs:
    %   dy  : Smoothed derivative estimate
    %   ema : Updated EMA value
    
    % Calculate smoothing factor from time constant
    alpha = 1 - exp(-dt ./ tau);
    
    % Update Exponential Moving Average
    ema = alpha .* y + (1 - alpha) .* ema_prev;
    
    % Compute derivative using finite difference on smoothed values
    dy = (ema - ema_prev) ./ dt;
end

== matlab function GNC2026W/PhaseSpace Camera Code/Use Hardware to Obtain States/Store BLACK Data/Subsystem2/Enabled Subsystem/MATLAB Function ==
  data: y input; dy output; dt input; tau input; ema_prev input; ema output
function [dy, ema] = realtime_derivative_ema(y, dt, tau, ema_prev)
    % Compute smoothed derivative using Exponential Moving Average
    %
    % Inputs:
    %   y        : Current measurement
    %   dt       : Time step
    %   tau      : Time constant for EMA filter (larger = more smoothing)
    %   ema_prev : Previous EMA value
    %
    % Outputs:
    %   dy  : Smoothed derivative estimate
    %   ema : Updated EMA value
    
    % Calculate smoothing factor from time constant
    alpha = 1 - exp(-dt ./ tau);
    
    % Update Exponential Moving Average
    ema = alpha .* y + (1 - alpha) .* ema_prev;
    
    % Compute derivative using finite difference on smoothed values
    dy = (ema - ema_prev) ./ dt;
end

== matlab function GNC2026W/PhaseSpace Camera Code/Use Hardware to Obtain States/Store BLUE Data/Calculate True Time Step/MATLAB Function ==
  data: dt input; dt_out output; dataRate input
function dt_out = CheckforInvalidTime(dt, dataRate)

    if dt <= 0

        dt_out = dataRate;

    else

        dt_out = dt;

    end


end

== matlab function GNC2026W/PhaseSpace Camera Code/Use Hardware to Obtain States/Store BLUE Data/Subsystem1/Enabled Subsystem/MATLAB Function ==
  data: y input; dy output; dt input; tau input; ema_prev input; ema output
function [dy, ema] = realtime_derivative_ema(y, dt, tau, ema_prev)
    % Compute smoothed derivative using Exponential Moving Average
    %
    % Inputs:
    %   y        : Current measurement
    %   dt       : Time step
    %   tau      : Time constant for EMA filter (larger = more smoothing)
    %   ema_prev : Previous EMA value
    %
    % Outputs:
    %   dy  : Smoothed derivative estimate
    %   ema : Updated EMA value
    
    % Calculate smoothing factor from time constant
    alpha = 1 - exp(-dt ./ tau);
    
    % Update Exponential Moving Average
    ema = alpha .* y + (1 - alpha) .* ema_prev;
    
    % Compute derivative using finite difference on smoothed values
    dy = (ema - ema_prev) ./ dt;
end

== matlab function GNC2026W/PhaseSpace Camera Code/Use Hardware to Obtain States/Store BLUE Data/Subsystem2/Enabled Subsystem/MATLAB Function ==
  data: y input; dy output; dt input; tau input; ema_prev input; ema output
function [dy, ema] = realtime_derivative_ema(y, dt, tau, ema_prev)
    % Compute smoothed derivative using Exponential Moving Average
    %
    % Inputs:
    %   y        : Current measurement
    %   dt       : Time step
    %   tau      : Time constant for EMA filter (larger = more smoothing)
    %   ema_prev : Previous EMA value
    %
    % Outputs:
    %   dy  : Smoothed derivative estimate
    %   ema : Updated EMA value
    
    % Calculate smoothing factor from time constant
    alpha = 1 - exp(-dt ./ tau);
    
    % Update Exponential Moving Average
    ema = alpha .* y + (1 - alpha) .* ema_prev;
    
    % Compute derivative using finite difference on smoothed values
    dy = (ema - ema_prev) ./ dt;
end

== matlab function GNC2026W/Simulate Plant Dynamics/RED and ARM Dynamics/RED Only/Dynamics Model for RED/MATLAB Function ==
  data: control_inputs input; x_ddot output; mRED parameter; IRED parameter

    function x_ddot = RED_dynamics(control_inputs, mRED, IRED)

        %#codegen
        % Fully define the size of x_ddot() for code generation:
        x_ddot     = zeros(3,1);

        % Extract the servicer model parameters from the model_param vector defined
        % in initialize.m:

        % Extract the control inputs from the control_input vector:
        Fx        = control_inputs(1);              % [N]
        Fy        = control_inputs(2);              % [N]
        Tz        = control_inputs(3);              % [N.m]

        % Calculate the state acceleration vector:
        x_ddot(1) = Fx/mRED;                      % [m/s^2]
        x_ddot(2) = Fy/mRED;                      % [m/s^2]
        x_ddot(3) = Tz/IRED;                      % [rad/s^2]

    end

== matlab function GNC2026W/PhaseSpace Camera Code/Use Hardware to Obtain States/Receive and Process Phasespace Data/Check for Sychronization (Updated)/MATLAB Function ==
  data: StartClock output; RedReceiving input; BlackReceiving input; BlueReceiving input; platformSelection parameter
function StartClock = CheckForSync(RedReceiving, BlackReceiving, BlueReceiving, platformSelection)
        
    StartClock = 0;
    
    if (platformSelection == 1)
        
        if RedReceiving ~= 0

            StartClock = 1;

        else

            StartClock = 0;

        end
        
    elseif (platformSelection == 2)
        
        if BlackReceiving ~= 0

            StartClock = 1;

        else

            StartClock = 0;

        end  
        
    elseif (platformSelection == 3)
        
        if RedReceiving ~= 0 && BlackReceiving ~=0

            StartClock = 1;

        else

            StartClock = 0;

        end    
        
    elseif (platformSelection == 4)
        
        if RedReceiving ~= 1 && BlackReceiving ~= 1

            StartClock = 1;

        else

            StartClock = 0;

        end
        
    elseif (platformSelection == 5)
        
        if RedReceiving ~= 1

            StartClock = 1;

        else

            StartClock = 0;

        end
        
    elseif (platformSelection == 6)
        
        if BlueReceiving ~= 1

            StartClock = 1;

        else

            StartClock = 0;

        end
        
    elseif (platformSelection == 7)
        
        if RedReceiving ~= 1 && BlueReceiving ~= 1

            StartClock = 1;

        else

            StartClock = 0;

        end
        
    elseif (platformSelection == 8)
        
        if RedReceiving ~= 1 && BlackReceiving ~= 1 && BlueReceiving ~= 1

            StartClock = 1;

        else

            StartClock = 0;

        end
        
    elseif (platformSelection == 9)
        
        if BlackReceiving ~= 1 && BlueReceiving ~= 1

            StartClock = 1;

        else

            StartClock = 0;

        end
                           
    elseif (platformSelection == 10)
        
        if RedReceiving ~= 1 && BlueReceiving ~= 1

            StartClock = 1;

        else

            StartClock = 0;

        end
        
    elseif (platformSelection == 11)
        
        if RedReceiving ~= 1 && BlackReceiving ~= 1 && BlueReceiving ~= 1

            StartClock = 1;

        else

            StartClock = 0;

        end
        
    end



end

== matlab function GNC2026W/PhaseSpace Camera Code/Use Hardware to Obtain States/Receive and Process Phasespace Data/Check for Sychronization (Updated)/MATLAB Function1 ==
  data: t1 input; t_min output; t2 input; t3 input
function t_min = MinNonZero(t1, t2, t3)

    t = [t1, t2, t3];

    t(t == 0 ) = NaN;
    [t_min,~] = min(t);

end

== matlab function GNC2026W/Simulate Plant Dynamics/RED and ARM Dynamics/RED + ARM/Calculated & Store Measured States/Subsystem5/Enabled Subsystem/MATLAB Function ==
  data: y input; dy output; dt input; tau input; ema_prev input; ema output
function [dy, ema] = realtime_derivative_ema(y, dt, tau, ema_prev)
    % Compute smoothed derivative using Exponential Moving Average
    %
    % Inputs:
    %   y        : Current measurement
    %   dt       : Time step
    %   tau      : Time constant for EMA filter (larger = more smoothing)
    %   ema_prev : Previous EMA value
    %
    % Outputs:
    %   dy  : Smoothed derivative estimate
    %   ema : Updated EMA value
    
    % Calculate smoothing factor from time constant
    alpha = 1 - exp(-dt ./ tau);
    
    % Update Exponential Moving Average
    ema = alpha .* y + (1 - alpha) .* ema_prev;
    
    % Compute derivative using finite difference on smoothed values
    dy = (ema - ema_prev) ./ dt;
end

== matlab function GNC2026W/Simulate Plant Dynamics/RED and ARM Dynamics/RED + ARM/Data @ Measurement Rate/Calculate True Time Step/MATLAB Function ==
  data: dt input; dt_out output; dataRate input
function dt_out = CheckforInvalidTime(dt, dataRate)

    if dt <= 0

        dt_out = dataRate;

    else

        dt_out = dt;

    end


end

== matlab function GNC2026W/PhaseSpace Camera Code/Use Hardware to Obtain States/Store BLACK Data/Simulated Noise  (HARDWARE)/BLK CoM to LAR ==
  data: r_T_I input; LARstates_I output
% Calculates position vector of LAR based on position vector of Target CoM 
function LARstates_I = fcn(r_T_I)

LARstates_I = r_T_I;

LAR_x = 0.145; % LAR offset in target BoF, m
th_T  = r_T_I(3);
C_IT  = [cos(th_T) -sin(th_T); sin(th_T) cos(th_T)]; % Target to inertial ref frame rotation matrix


LARstates_I(1:2) = r_T_I(1:2) + C_IT*[LAR_x;0];

end

== matlab function GNC2026W/Simulate Plant Dynamics/BLACK Dynamics/Simulated Noise /CV Noise ==
  data: u input; y output
% Noise simulation

% Ally Colla
% Chris El-Asmar

function y = CVnoise (u)
% u = black true state + gaussian white noise 
% y = expected computer vision noise


% Tunable Parameters
quantization = 0.0001;  % amplitude of steps
spikeprob = 0.5; % probability of spikes happening
spikemag  = 0.1;  % magnitude of spikes ~ 10 cm

% Randomize spikes
if rand < spikeprob && spikemag < 1
    u = u + spikemag * (2*rand-1); % spikes with different magnitudes between -1 and 1
end

% Quantization 
y = quantization * round(u/quantization); % scale the signal


end

== matlab function GNC2026W/2 - Guidance/Custom PPL (RED)/MATLAB Function4 ==
  data: blkSTATES input; q_des output; L0 input
function q_des = PPL(blkSTATES, L0)

% Nimish Dhawan
% Sukriti Kumar
% 2025

%%%%%%%%%%%%%%%%%%%%%%%%%%%%%%%%%%%%%%%%%%%%%%%%%%%%%%%%%%%%%%%%%%%%%%%%%
% Input(s)
%%%%%%%%%%%%%%%%%%%%%%%%%%%%%%%%%%%%%%%%%%%%%%%%%%%%%%%%%%%%%%%%%%%%%%%%%
% blkSTATES (9x1): [pose(3x1); velocity(3x1); acceleration(3x1)] of target
% L0 (1x1)       : distance from chaser to target

%%%%%%%%%%%%%%%%%%%%%%%%%%%%%%%%%%%%%%%%%%%%%%%%%%%%%%%%%%%%%%%%%%%%%%%%%
% Output(s)
%%%%%%%%%%%%%%%%%%%%%%%%%%%%%%%%%%%%%%%%%%%%%%%%%%%%%%%%%%%%%%%%%%%%%%%%%
% q_des (9x1): desired chaser pose [pose(3x1); velocity(3x1); acceleration(3x1)]

q_des = zeros(9,1);

x           = blkSTATES(1);
y           = blkSTATES(2);
theta       = blkSTATES(3);
x_dot       = blkSTATES(4);
y_dot       = blkSTATES(5);
theta_dot   = blkSTATES(6);
x_ddot      = 0;
y_ddot      = 0;
theta_ddot  = 0;

q_des(1) = x + L0*cos(theta);
q_des(2) = y + L0*sin(theta);
q_des(3) = theta + pi;
q_des(4) = x_dot - L0*theta_dot*sin(theta);
q_des(5) = y_dot + L0*theta_dot*cos(theta);
q_des(6) = theta_dot;
q_des(7) = x_ddot - theta_ddot*L0*sin(theta) - theta_dot^2*L0*cos(theta);
q_des(8) = y_ddot + theta_ddot*L0*cos(theta) - theta_dot^2*L0*sin(theta);
q_des(9) = theta_ddot;


end

== matlab function GNC2026W/PhaseSpace Camera Code/Use Hardware to Obtain States/Store BLACK Data/Simulated Noise  (HARDWARE)/CV Noise ==
  data: u input; y output
% Noise simulation

% Ally Colla
% Chris El-Asmar

function y = CVnoise (u)
% u = black true state + gaussian white noise 
% y = expected computer vision noise


% Tunable Parameters
quantization = 0.0001;  % amplitude of steps
spikeprob = 0.5; % probability of spikes happening
spikemag  = 0.1;  % magnitude of spikes ~ 10 cm

% Randomize spikes
if rand < spikeprob && spikemag < 1
    u = u + spikemag * (2*rand-1); % spikes with different magnitudes between -1 and 1
end

% Quantization 
y = quantization * round(u/quantization); % scale the signal


end

== matlab function GNC2026W/1 - Experiment Logic/Phase #3: Experiment/Sub-Phase #2 /Red Control Logic/First Fit Detector ==
  data: cmd output; isValid input; filterConfidence input
function cmd  = firstfit(isValid, filterConfidence)

persistent counter firstfit prev phase
if isempty(counter)
    counter  = 0; 
    firstfit = 0;
    prev     = 0;
    phase = 0;
end

% Checking for first fit of the ellipse
if isValid == 1 && firstfit == 0
    firstfit = 1;
end

% Waiting for 5 continuous valid readings
if firstfit == 1 && isValid == 1 && prev == 1
    if counter < 5
        % Hold position until 5 consecutive isValid = 1 are recorded
        phase = 0;
        % ctrlmode = 2;
        % pathplan = 2;
    elseif counter > 5 && filterConfidence == 0
        % Initiate filter after 5 consecutive isValid are recorded
        phase = 1;
        % ctrlmode = 2;
        % pathplan = 2;
    elseif counter > 5 && filterConfidence == 1
        % Start moving once the filter has converged
        phase = 2;
        % ctrlmode = 3;
        % pathplan = 1;
    end

    % Incrementing counter if there are two consecutive isValid = 1
    counter = counter+1; 
else
    if counter < 5
        % Hold position
        phase = 3;
        % ctrlmode = 2;
        % pathplan = 2;
    
        % Counter gets reset to 0 if isValid is not consecutively 1 at least
        % three times
        counter  = 0;
    elseif counter > 5 && filterConfidence == 0
        % If there is a frame drop and the filter has not converged yet,
        % hold position
        phase = 4;
        % ctrlmode = 2;
        % pathplan = 2;
    elseif counter > 5 && filterConfidence == 1
        % If there is a frame drop and filter has converged, trust the
        % estimates and move
        phase = 5;
        % ctrlmode = 3;
        % pathplan = 1;
    end
end

% Storing isValid value in prev
prev = isValid;
cmd = phase;


end

== matlab function GNC2026W/Data Logger Subsystem/Separation/MATLAB Function ==
  data: RED_path input; L output; BLACK_path input
function L = fcn(RED_path, BLACK_path)

    xc  = RED_path(1);  
    yc  = RED_path(2);
    xt  = BLACK_path(1); 
    yt  = BLACK_path(2);

    L  = sqrt((yc - yt)^2 + (xc - xt)^2);

end

== matlab function GNC2026W/3 - Control/Custom Control (RED)/Unwrap1/MATLAB Function ==
  data: u input; y output; u_pre input; y_pre input; u_next output
function [y, u_next] = fcn(u, u_pre, y_pre)

% Nimish Dhawan 2025
% Carleton University

%%%%%%%%%%%%%%%%%%%%%%%%%%%%%%%%%%%%%%%%%%%%%%%%%%%%%%%%%%%%%%%%%%%%%%%%%
% Inputs
%%%%%%%%%%%%%%%%%%%%%%%%%%%%%%%%%%%%%%%%%%%%%%%%%%%%%%%%%%%%%%%%%%%%%%%%%
% u (rad)       : current wrapped angle
% u_pre (rad)   : previous wrapped angle
% y_pre (rad)   : previous unwrapped angle

%%%%%%%%%%%%%%%%%%%%%%%%%%%%%%%%%%%%%%%%%%%%%%%%%%%%%%%%%%%%%%%%%%%%%%%%%
% Output
%%%%%%%%%%%%%%%%%%%%%%%%%%%%%%%%%%%%%%%%%%%%%%%%%%%%%%%%%%%%%%%%%%%%%%%%%
% y (rad)       : unwrapped angle
% u_next (rad)  : next wrapped angle

x = mod((u-u_pre)+pi, 2*pi) - pi;

y = y_pre + x;
u_next = u;

end

== matlab function GNC2026W/3 - Control/Custom Control (RED)/Unwrap/Unwrap/MATLAB Function ==
  data: u input; y output; u_pre input; y_pre input; u_next output
function [y, u_next] = fcn(u, u_pre, y_pre)

% Nimish Dhawan 2025
% Carleton University

%%%%%%%%%%%%%%%%%%%%%%%%%%%%%%%%%%%%%%%%%%%%%%%%%%%%%%%%%%%%%%%%%%%%%%%%%
% Inputs
%%%%%%%%%%%%%%%%%%%%%%%%%%%%%%%%%%%%%%%%%%%%%%%%%%%%%%%%%%%%%%%%%%%%%%%%%
% u (rad)       : current wrapped angle
% u_pre (rad)   : previous wrapped angle
% y_pre (rad)   : previous unwrapped angle

%%%%%%%%%%%%%%%%%%%%%%%%%%%%%%%%%%%%%%%%%%%%%%%%%%%%%%%%%%%%%%%%%%%%%%%%%
% Output
%%%%%%%%%%%%%%%%%%%%%%%%%%%%%%%%%%%%%%%%%%%%%%%%%%%%%%%%%%%%%%%%%%%%%%%%%
% y (rad)       : unwrapped angle
% u_next (rad)  : next wrapped angle

x = mod((u-u_pre)+pi, 2*pi) - pi;

y = y_pre + x;
u_next = u;

end

== matlab function GNC2026W/PhaseSpace Camera Code/Use Hardware to Obtain States/Store BLACK Data/Simulated Noise  (HARDWARE)/Inertial to Camera Frame (HARDWARE) ==
  data: r_C input; r_REL output; r_T input
% Rotation matrix to go from inertial to relative
function r_REL = CBI(r_C, r_T)
l_cam_x    = 0.125; %m, offset in x from origin of Red, left camera
l_cam_y    = 0.03; %m, offset in y from origin of Red, left camera
th_C       = r_C(3);
th_T       = r_T(3);
d_xy       = r_T(1:2) - r_C(1:2);
C_CI       = [cos(th_C) sin(th_C); -sin(th_C) cos(th_C)]; % Chaser to inertial ref frame rotation matrix
r_REL      = [C_CI*d_xy; th_T - th_C];
r_REL(1:2) = r_REL(1:2) - [l_cam_x; l_cam_y];
end

== matlab function GNC2026W/3 - Control/Custom Control (RED)/MATLAB Function2 ==
  data: REDact input; e output; REDdes input; thREL input; baseRate parameter; lambda output; lambdaFirstOrder output
function [e, lambda, lambdaFirstOrder] = err(REDact, REDdes, thREL, baseRate)

% Nimish Dhawan

%%%%%%%%%%%%%%%%%%%%%%%%%%%%%%%%%%%%%%%%%%%%%%%%%%%%%%%%%%%%%%%%%%%%%%%%%
% Input(s)
%%%%%%%%%%%%%%%%%%%%%%%%%%%%%%%%%%%%%%%%%%%%%%%%%%%%%%%%%%%%%%%%%%%%%%%%%


%%%%%%%%%%%%%%%%%%%%%%%%%%%%%%%%%%%%%%%%%%%%%%%%%%%%%%%%%%%%%%%%%%%%%%%%%
% Output(s)
%%%%%%%%%%%%%%%%%%%%%%%%%%%%%%%%%%%%%%%%%%%%%%%%%%%%%%%%%%%%%%%%%%%%%%%%%

persistent l1 l2 

if isempty(l1)
    l1 = 0;
    l2 = 0;
end

% Calculating line of sight angular velocity and acceleration
lambda = estLambda(thREL, baseRate);

e = [REDact; zeros(3,1)] - REDdes;

% Overwriting the angle error with new line of sight angle
e(3) = -lambda(1);
e(6) = -lambda(2);
e(9) = -lambda(3);

% First order approximation calculation
l = thREL;
lDot = (l-l1)/baseRate;
lDdot = (l-2*l1+l2)/baseRate;

lambdaFirstOrder = [l; lDot; lDdot];

l2 = l1;
l1 = l;


end
%%
function [lambda_est] = estLambda(meas, dt)

persistent x P

if isempty(x)
    x = [meas; 0; 0];
    P = zeros(3,3);
end

Q  = 1e-3*eye(3);
% R  = 1e-09; 

% Propagate
F = [1 dt 0; 0 1 dt; 0 0 0];

x_minus = F*x;
P_minus = F*P*F' + Q;

% Update
H   = [1 0 0];
res = meas - H*x_minus;
S   = (H*P_minus*H');
K   = P_minus*H' / S;

x = x_minus + K*res;
P = (eye(3)-K*H)*P_minus;

lambda_est = x;

end

== matlab function GNC2026W/Thruster Control Code/Change BLACK Behavior/Calculate Duty Cycle/Generate Initial Guess/MATLAB Function ==
  data: H output; thruster_dist2CG_BLACK parameter; F_thrusters_BLACK parameter
function H = MakeH(thruster_dist2CG_BLACK,F_thrusters_BLACK)

    Vec1 = [ -1
             -1
              0 
              0
              1
              1
              0
              0 ];
          
    Vec2 = [  0
              0
              1
              1
              0
              0
             -1
             -1 ];
         
    Vec3 = thruster_dist2CG_BLACK./1000;
    
    Mat1 = [Vec1, Vec2, Vec3]';
    
    Mat2 = diag((F_thrusters_BLACK./2));
    
    H    = Mat1*Mat2;

end

== matlab function GNC2026W/3 - Control/Custom Control (RED)/MATLAB Function3 ==
  data: F_c output; A_c input; F_u input; error input; alpha parameter; gamma parameter; Mc_inv parameter
function F_c = fcn(A_c, F_u, error, alpha, gamma, Mc_inv)

% Nimish Dhawan

%%%%%%%%%%%%%%%%%%%%%%%%%%%%%%%%%%%%%%%%%%%%%%%%%%%%%%%%%%%%%%%%%%%%%%%%%
% Input(s)
%%%%%%%%%%%%%%%%%%%%%%%%%%%%%%%%%%%%%%%%%%%%%%%%%%%%%%%%%%%%%%%%%%%%%%%%%
% alpha (3x3): derivative gain
% gamma (3x3): proportional gain
% error (9x1): actual - desired chaser pose
% M_inv (3x3): mass matrix inverse
% F_u (3x1)  : unconstrained forces
% A_c (3x3)

%%%%%%%%%%%%%%%%%%%%%%%%%%%%%%%%%%%%%%%%%%%%%%%%%%%%%%%%%%%%%%%%%%%%%%%%%
% Output(s)
%%%%%%%%%%%%%%%%%%%%%%%%%%%%%%%%%%%%%%%%%%%%%%%%%%%%%%%%%%%%%%%%%%%%%%%%%
% F_c (3x1): control forces in N

b_c = - error(7:9) - alpha * error(4:6) - gamma * error(1:3);

F_c = A_c' * pinv(A_c*Mc_inv*A_c') * (b_c - A_c*Mc_inv*F_u);

end
%%
function [alpha, gamma] = gainscheduler(theta, Kp, Kd)

theta = theta - pi;
threshold = deg2rad(25);
alpha = Kp;
gamma = Kd;

if cos(theta) >= cos(threshold)
    alpha(3) = 5;
    gamma(3) = 2.5;

end

end

== matlab function GNC2026W/Simulate Plant Dynamics/RED and ARM Dynamics/RED Only/Calculated & Store Measured States/Subsystem1/Enabled Subsystem/MATLAB Function ==
  data: y input; dy output; dt input; tau input; ema_prev input; ema output
function [dy, ema] = realtime_derivative_ema(y, dt, tau, ema_prev)
    % Compute smoothed derivative using Exponential Moving Average
    %
    % Inputs:
    %   y        : Current measurement
    %   dt       : Time step
    %   tau      : Time constant for EMA filter (larger = more smoothing)
    %   ema_prev : Previous EMA value
    %
    % Outputs:
    %   dy  : Smoothed derivative estimate
    %   ema : Updated EMA value
    
    % Calculate smoothing factor from time constant
    alpha = 1 - exp(-dt ./ tau);
    
    % Update Exponential Moving Average
    ema = alpha .* y + (1 - alpha) .* ema_prev;
    
    % Compute derivative using finite difference on smoothed values
    dy = (ema - ema_prev) ./ dt;
end

== matlab function GNC2026W/Thruster Control Code/Change BLACK Behavior/Calculate Duty Cycle/Rotate Forces to Inertial/Create Rotation Matrix ==
  data: Rz input; C_Ib output
function C_Ib = RotateFrame(Rz)

C_bI = [  cos(Rz) sin(Rz)
         -sin(Rz) cos(Rz) ];

C_Ib = inv(C_bI);

end
